simulink model "Model"  (R2024b)
settings: Solver=VariableStepAuto  StartTime=0.0  StopTime=30  MaxStep=0.001  RelTol=1e-4
PostLoadFcn:
  | SIM_setup
values from neighbouring files (symbols this model uses):
  A = 1.1    [RT14e_Parameters.m]    (also in RT15e_Parameters.m = 1.088; RT15evo_Parameters.m = 1.088; SIM_setup.m = 1.12)
  Aero_balance = 55    [RT14e_Parameters.m]    (also in RT15e_Parameters.m; RT15evo_Parameters.m; SIM_setup.m = 0.55)
  air_density = 1.29    [SIM_setup.m]
  Br_coef_of_friction_F = 0.33    [RT14e_Parameters.m]    (also in RT15e_Parameters.m; RT15evo_Parameters.m; SIM_setup.m = 0.25)
  Br_coef_of_friction_R = 0.33    [RT14e_Parameters.m]    (also in RT15e_Parameters.m; RT15evo_Parameters.m; SIM_setup.m = 0.25)
  Br_pistons_area_F = 3617.26/1e6    (= 0.00361726)    [RT14e_Parameters.m]    (also in RT15e_Parameters.m; RT15evo_Parameters.m; SIM_setup.m)
  Br_pistons_area_R = 2026.83/1e6    (= 0.00202683)    [RT14e_Parameters.m]    (also in RT15e_Parameters.m; RT15evo_Parameters.m; SIM_setup.m)
  Cd = 1.387    [SIM_setup.m]
  Cl = 3.299    [SIM_setup.m]
  CoG_z = 0.35    [RT14e_Parameters.m]    (also in RT15e_Parameters.m = 0.28495; RT15evo_Parameters.m = 0.28495; SIM_setup.m = 0.328)
  Default_Fz_F = g*(Mass*(Lr/Wheelbase))    [RT14e_Parameters.m]    (also in RT15e_Parameters.m; RT15evo_Parameters.m; SIM_setup.m = 608.22)
  Default_Fz_R = g*(Mass*(Lf/Wheelbase))    [RT14e_Parameters.m]    (also in RT15e_Parameters.m; RT15evo_Parameters.m; SIM_setup.m = 774.99)
  Effective_br_disk_r_F = 0.0905    [RT14e_Parameters.m]    (also in RT15e_Parameters.m; RT15evo_Parameters.m; SIM_setup.m)
  Effective_br_disk_r_R = 0.0895    [RT14e_Parameters.m]    (also in RT15e_Parameters.m; RT15evo_Parameters.m; SIM_setup.m)
  Fx = Data_Fx(2:end,3:end)    [RT14e_Parameters.m]    (also in RT15e_Parameters.m; RT15evo_Parameters.m; SIM_setup.m = Data_Fx(2:end,2:end))
  Fy = Data_Fy(2:end,3:end)    [RT14e_Parameters.m]    (also in RT15e_Parameters.m; RT15evo_Parameters.m; SIM_setup.m = Data_Fy(2:end,2:end))
  Fz = Data_Fy(2:end,2)    [RT14e_Parameters.m]    (also in RT15e_Parameters.m; RT15evo_Parameters.m; SIM_setup.m = Data_Fy(2:end,1))
  Half_track = 0.6    [SIM_setup.m]
  Iz_wehicle = 120    [RT14e_Parameters.m]    (also in RT15e_Parameters.m; RT15evo_Parameters.m; SIM_setup.m)
  Iz_wheel = 0.15    [RT14e_Parameters.m]    (also in RT15e_Parameters.m; RT15evo_Parameters.m; SIM_setup.m)
  Lateral_load_transfer_distribution = 0.55    [SIM_setup.m]
  Lf = Wheelbase - CoG_x    (= 0.77)    [RT14e_Parameters.m]    (also in RT15e_Parameters.m = 0.7504; RT15evo_Parameters.m = 0.7504; SIM_setup.m)
  Lr = Wheelbase - Lf    (= 0.755)    [RT14e_Parameters.m]    (also in RT15e_Parameters.m = 0.7746; RT15evo_Parameters.m = 0.7746; SIM_setup.m)
  Mass = Vehicle_mass + Driver_mass    (= 290)    [RT14e_Parameters.m]    (also in RT15e_Parameters.m = 265; RT15evo_Parameters.m; SIM_setup.m = 300)
  Max_Torque = 29.1    [SIM_setup.m]
  RB_torque_setting_1 = -2    [RT14e_Parameters.m]    (also in RT15e_Parameters.m; RT15evo_Parameters.m; SIM_setup.m)
  RB_torque_setting_10 = -20    [RT14e_Parameters.m]    (also in RT15e_Parameters.m; RT15evo_Parameters.m; SIM_setup.m)
  RB_torque_setting_2 = -4    [RT14e_Parameters.m]    (also in RT15e_Parameters.m; RT15evo_Parameters.m; SIM_setup.m)
  RB_torque_setting_3 = -6    [RT14e_Parameters.m]    (also in RT15e_Parameters.m; RT15evo_Parameters.m; SIM_setup.m)
  RB_torque_setting_4 = -8    [RT14e_Parameters.m]    (also in RT15e_Parameters.m; RT15evo_Parameters.m; SIM_setup.m)
  RB_torque_setting_5 = -10    [RT14e_Parameters.m]    (also in RT15e_Parameters.m; RT15evo_Parameters.m; SIM_setup.m)
  RB_torque_setting_6 = -12    [RT14e_Parameters.m]    (also in RT15e_Parameters.m; RT15evo_Parameters.m; SIM_setup.m)
  RB_torque_setting_7 = -14    [RT14e_Parameters.m]    (also in RT15e_Parameters.m; RT15evo_Parameters.m; SIM_setup.m)
  RB_torque_setting_8 = -16    [RT14e_Parameters.m]    (also in RT15e_Parameters.m; RT15evo_Parameters.m; SIM_setup.m)
  RB_torque_setting_9 = -18    [RT14e_Parameters.m]    (also in RT15e_Parameters.m; RT15evo_Parameters.m; SIM_setup.m)
  SA = Data_Fy(1,3:end)    [RT14e_Parameters.m]    (also in RT15e_Parameters.m; RT15evo_Parameters.m; SIM_setup.m = Data_Fy(1,2:end))
  SR = Data_Fx(1,3:end)    [RT14e_Parameters.m]    (also in RT15e_Parameters.m; RT15evo_Parameters.m; SIM_setup.m = Data_Fx(1,2:end))
  start_time = 182    [SIM_setup.m]
  start_velocity = Xsens_MTI_670_vel.Value(find(Xsens_MTI_670_vel.Time > start_time, 1)) * 1000 / 3600    [SIM_setup.m]
  Steering_angle_table = [0 9.9 19.9 30.14 40.57 51.05 61.29 70.87 79.38 91.9]    [SIM_setup.m]
  Steering_ratio_table = [3.25 3.24 3.23 3.20 3.16 3.10 3.04 2.97 2.90 2.77]    [SIM_setup.m]
  Tire_radius = 0.203    [RT14e_Parameters.m]    (also in RT15e_Parameters.m; RT15evo_Parameters.m; SIM_setup.m)
  Torque_limit_2 = Motor_maximum_torque*0.2    (= 5.82)    [RT14e_Parameters.m]    (also in RT15e_Parameters.m; RT15evo_Parameters.m; SIM_setup.m)
  Torque_limit_3 = Motor_maximum_torque*0.3    (= 8.73)    [RT14e_Parameters.m]    (also in RT15e_Parameters.m; RT15evo_Parameters.m; SIM_setup.m)
  Torque_limit_4 = Motor_maximum_torque*0.4    (= 11.64)    [RT14e_Parameters.m]    (also in RT15e_Parameters.m; RT15evo_Parameters.m; SIM_setup.m)
  Torque_limit_5 = Motor_maximum_torque*0.5    (= 14.55)    [RT14e_Parameters.m]    (also in RT15e_Parameters.m; RT15evo_Parameters.m; SIM_setup.m)
  Torque_limit_6 = Motor_maximum_torque*0.6    (= 17.46)    [RT14e_Parameters.m]    (also in RT15e_Parameters.m; RT15evo_Parameters.m; SIM_setup.m)
  Torque_limit_7 = Motor_maximum_torque*0.7    (= 20.37)    [RT14e_Parameters.m]    (also in RT15e_Parameters.m; RT15evo_Parameters.m; SIM_setup.m)
  Torque_limit_8 = Motor_maximum_torque*0.8    (= 23.28)    [RT14e_Parameters.m]    (also in RT15e_Parameters.m; RT15evo_Parameters.m; SIM_setup.m)
  Torque_limit_9 = 29.1    [RT14e_Parameters.m]    (also in RT15e_Parameters.m; RT15evo_Parameters.m; SIM_setup.m)
  Torque_limit_max = Motor_maximum_torque    (= 29.1)    [RT14e_Parameters.m]    (also in RT15e_Parameters.m; RT15evo_Parameters.m; SIM_setup.m)
  Torque_limit_min = Motor_maximum_torque*0.1    (= 2.91)    [RT14e_Parameters.m]    (also in RT15e_Parameters.m; RT15evo_Parameters.m; SIM_setup.m)
  Transmission_gear_ratio = 12.9    [SIM_setup.m]
  TV_RB_understeer_gradient_1 = -0.5    [RT14e_Parameters.m]    (also in RT15e_Parameters.m; RT15evo_Parameters.m; SIM_setup.m)
  TV_RB_understeer_gradient_10 = 0.005    [RT14e_Parameters.m]    (also in RT15e_Parameters.m; RT15evo_Parameters.m; SIM_setup.m)
  TV_RB_understeer_gradient_2 = -0.1    [RT14e_Parameters.m]    (also in RT15e_Parameters.m; RT15evo_Parameters.m; SIM_setup.m)
  TV_RB_understeer_gradient_3 = 0.08    [RT14e_Parameters.m]    (also in RT15e_Parameters.m; RT15evo_Parameters.m; SIM_setup.m)
  TV_RB_understeer_gradient_4 = 0.06    [RT14e_Parameters.m]    (also in RT15e_Parameters.m; RT15evo_Parameters.m; SIM_setup.m)
  TV_RB_understeer_gradient_5 = 0.05    [RT14e_Parameters.m]    (also in RT15e_Parameters.m; RT15evo_Parameters.m; SIM_setup.m)
  TV_RB_understeer_gradient_6 = 0.04    [RT14e_Parameters.m]    (also in RT15e_Parameters.m; RT15evo_Parameters.m; SIM_setup.m)
  TV_RB_understeer_gradient_7 = 0.03    [RT14e_Parameters.m]    (also in RT15e_Parameters.m; RT15evo_Parameters.m; SIM_setup.m)
  TV_RB_understeer_gradient_8 = 0.02    [RT14e_Parameters.m]    (also in RT15e_Parameters.m; RT15evo_Parameters.m; SIM_setup.m)
  TV_RB_understeer_gradient_9 = 0.01    [RT14e_Parameters.m]    (also in RT15e_Parameters.m; RT15evo_Parameters.m; SIM_setup.m)
  TV_understeer_gradient_1 = -0.5    [RT14e_Parameters.m]    (also in RT15e_Parameters.m; RT15evo_Parameters.m; SIM_setup.m)
  TV_understeer_gradient_10 = 0.002    [RT14e_Parameters.m]    (also in RT15e_Parameters.m; RT15evo_Parameters.m; SIM_setup.m)
  TV_understeer_gradient_2 = -0.1    [RT14e_Parameters.m]    (also in RT15e_Parameters.m; RT15evo_Parameters.m; SIM_setup.m)
  TV_understeer_gradient_3 = 0.06    [RT14e_Parameters.m]    (also in RT15e_Parameters.m; RT15evo_Parameters.m; SIM_setup.m)
  TV_understeer_gradient_4 = 0.05    [RT14e_Parameters.m]    (also in RT15e_Parameters.m; RT15evo_Parameters.m; SIM_setup.m)
  TV_understeer_gradient_5 = 0.04    [RT14e_Parameters.m]    (also in RT15e_Parameters.m; RT15evo_Parameters.m; SIM_setup.m)
  TV_understeer_gradient_6 = 0.03    [RT14e_Parameters.m]    (also in RT15e_Parameters.m; RT15evo_Parameters.m; SIM_setup.m)
  TV_understeer_gradient_7 = 0.02    [RT14e_Parameters.m]    (also in RT15e_Parameters.m; RT15evo_Parameters.m; SIM_setup.m)
  TV_understeer_gradient_8 = 0.01    [RT14e_Parameters.m]    (also in RT15e_Parameters.m; RT15evo_Parameters.m; SIM_setup.m)
  TV_understeer_gradient_9 = 0.005    [RT14e_Parameters.m]    (also in RT15e_Parameters.m; RT15evo_Parameters.m; SIM_setup.m)
  Wheel_base = 1.525    [SIM_setup.m]
  Wheel_rolling_resistance = 0.055    [RT14e_Parameters.m]    (also in RT15e_Parameters.m; RT15evo_Parameters.m; SIM_setup.m)
undefined symbols (not defined in the file or in its folder): Actual_Torque_Value_RL, Actual_Torque_Value_RR, aero_balance, APPS, Brake_Pressure_Front, Brake_Pressure_Rear, lateral_load_transfer_distribution, Steering_position, tire_radius, wheel_base, Xsens_MTI_670_accX, Xsens_MTI_670_accY, Xsens_MTI_670_gyrZ, Xsens_MTI_670_vel, Xsens_Yaw_Rate__deg_s_
libraries: simulink x20, simulink_extras x7, dspstat3 x4, slpidlib x1, slrealtimeloglib x1
(part 4 of 4)

== system Model/Drivetrain/TV Algorithm/Torque Vectoring/RB Yaw Rate Calculation/Understeer Gradeint Selection/Switch Case Action Subsystem20 ==
  Action Port : ActionPort  ActionPortLabel=case [ 9 ]:
  Constant : Constant  Value=TV_RB_understeer_gradient_9
  Out2 : Outport
  wires:
  Constant/1 -> Out2/1

== system Model/Drivetrain/TV Algorithm/Torque Vectoring/RB Yaw Rate Calculation/Understeer Gradeint Selection/Switch Case Action Subsystem21 ==
  Action Port : ActionPort  ActionPortLabel=case [ 10 ]:
  Constant : Constant  Value=TV_RB_understeer_gradient_10
  Out1 : Outport
  wires:
  Constant/1 -> Out1/1

== system Model/Drivetrain/TV Algorithm/Torque Vectoring/Yaw Rate Calculation/Understeer Gradeint Selection/Switch Case Action Subsystem ==
  Vehicle Speed [km/h] : Inport
  Action Port : ActionPort  ActionPortLabel=case [ 1 ]:
  1-D Lookup Table : Lookup_n-D  NumberOfTableDimensions=1  BreakpointsForDimension1=[25;30;35;40;45;50;55;60;65;70;75;80]  Table=[0.03;0.06;0.08;0.1;0.12;0.15;0.22;0.3;0.35;0.42;0.48;0.55]  InternalRulePriority=Speed  RndMeth=Simplest
  Saturation : Saturate  UpperLimit=80  LowerLimit=25
  Saturation1 : Saturate  UpperLimit=0.55  LowerLimit=0.03
  Out1 : Outport
  wires:
  1-D Lookup Table/1 -> Saturation1/1
  Saturation1/1 -> Out1/1
  Vehicle Speed [km/h]/1 -> Saturation/1
  Saturation/1 -> 1-D Lookup Table/1

== system Model/Drivetrain/TV Algorithm/Torque Vectoring/Yaw Rate Calculation/Understeer Gradeint Selection/Switch Case Action Subsystem1 ==
  Vehicle Speed [km/h] : Inport
  Action Port : ActionPort  ActionPortLabel=case [ 2 ]:
  1-D Lookup Table : Lookup_n-D  NumberOfTableDimensions=1  BreakpointsForDimension1=[25;30;35;40;45;50;55;60;65;70;75;80]  Table=[0.02;0.04;0.06;0.08;0.1;0.14;0.16;0.2;0.25;0.32;0.38;0.45]  InternalRulePriority=Speed  RndMeth=Simplest
  Saturation : Saturate  UpperLimit=80  LowerLimit=25
  Saturation1 : Saturate  UpperLimit=0.45  LowerLimit=0.02
  Out1 : Outport
  wires:
  Vehicle Speed [km/h]/1 -> Saturation/1
  Saturation/1 -> 1-D Lookup Table/1
  1-D Lookup Table/1 -> Saturation1/1
  Saturation1/1 -> Out1/1

== system Model/Drivetrain/TV Algorithm/Torque Vectoring/Yaw Rate Calculation/Understeer Gradeint Selection/Switch Case Action Subsystem10 ==
  Vehicle Speed [km/h] : Inport
  Action Port : ActionPort  ActionPortLabel=default:
  1-D Lookup Table : Lookup_n-D  NumberOfTableDimensions=1  BreakpointsForDimension1=[25;30;35;40;45;50;55;60;65;70;75;80]  Table=[0.003;0.005;0.008;0.01;0.03;0.05;0.08;0.12;0.15;0.18;0.25;0.3]  InternalRulePriority=Speed  RndMeth=Simplest
  Saturation : Saturate  UpperLimit=80  LowerLimit=25
  Saturation1 : Saturate  UpperLimit=0.3  LowerLimit=0.001
  Out1 : Outport
  wires:
  1-D Lookup Table/1 -> Saturation1/1
  Vehicle Speed [km/h]/1 -> Saturation/1
  Saturation1/1 -> Out1/1
  Saturation/1 -> 1-D Lookup Table/1

== system Model/Drivetrain/TV Algorithm/Torque Vectoring/Yaw Rate Calculation/Understeer Gradeint Selection/Switch Case Action Subsystem11 ==
  Action Port : ActionPort  ActionPortLabel=case [ 1 ]:
  Constant1 : Constant  Value=TV_understeer_gradient_1
  Out1 : Outport
  wires:
  Constant1/1 -> Out1/1

== system Model/Drivetrain/TV Algorithm/Torque Vectoring/Yaw Rate Calculation/Understeer Gradeint Selection/Switch Case Action Subsystem12 ==
  Action Port : ActionPort  ActionPortLabel=case [ 2 ]:
  Constant : Constant  Value=TV_understeer_gradient_2
  Out2 : Outport
  wires:
  Constant/1 -> Out2/1

== system Model/Drivetrain/TV Algorithm/Torque Vectoring/Yaw Rate Calculation/Understeer Gradeint Selection/Switch Case Action Subsystem13 ==
  Action Port : ActionPort  ActionPortLabel=default:
  Constant : Constant  Value=TV_understeer_gradient_8
  Out2 : Outport
  wires:
  Constant/1 -> Out2/1

== system Model/Drivetrain/TV Algorithm/Torque Vectoring/Yaw Rate Calculation/Understeer Gradeint Selection/Switch Case Action Subsystem14 ==
  Action Port : ActionPort  ActionPortLabel=case [ 3 ]:
  Constant1 : Constant  Value=TV_understeer_gradient_3
  Out1 : Outport
  wires:
  Constant1/1 -> Out1/1

== system Model/Drivetrain/TV Algorithm/Torque Vectoring/Yaw Rate Calculation/Understeer Gradeint Selection/Switch Case Action Subsystem15 ==
  Action Port : ActionPort  ActionPortLabel=case [ 4 ]:
  Constant : Constant  Value=TV_understeer_gradient_4
  Out2 : Outport
  wires:
  Constant/1 -> Out2/1

== system Model/Drivetrain/TV Algorithm/Torque Vectoring/Yaw Rate Calculation/Understeer Gradeint Selection/Switch Case Action Subsystem16 ==
  Action Port : ActionPort  ActionPortLabel=case [ 5 ]:
  Constant : Constant  Value=TV_understeer_gradient_5
  Out1 : Outport
  wires:
  Constant/1 -> Out1/1

== system Model/Drivetrain/TV Algorithm/Torque Vectoring/Yaw Rate Calculation/Understeer Gradeint Selection/Switch Case Action Subsystem17 ==
  Action Port : ActionPort  ActionPortLabel=case [ 6 ]:
  Constant : Constant  Value=TV_understeer_gradient_6
  Out2 : Outport
  wires:
  Constant/1 -> Out2/1

== system Model/Drivetrain/TV Algorithm/Torque Vectoring/Yaw Rate Calculation/Understeer Gradeint Selection/Switch Case Action Subsystem18 ==
  Action Port : ActionPort  ActionPortLabel=case [ 7 ]:
  Constant : Constant  Value=TV_understeer_gradient_7
  Out1 : Outport
  wires:
  Constant/1 -> Out1/1

== system Model/Drivetrain/TV Algorithm/Torque Vectoring/Yaw Rate Calculation/Understeer Gradeint Selection/Switch Case Action Subsystem19 ==
  Action Port : ActionPort  ActionPortLabel=case [ 8 ]:
  Constant : Constant  Value=TV_understeer_gradient_8
  Out2 : Outport
  wires:
  Constant/1 -> Out2/1

== system Model/Drivetrain/TV Algorithm/Torque Vectoring/Yaw Rate Calculation/Understeer Gradeint Selection/Switch Case Action Subsystem2 ==
  Vehicle Speed [km/h] : Inport
  Action Port : ActionPort  ActionPortLabel=case [ 3 ]:
  1-D Lookup Table1 : Lookup_n-D  NumberOfTableDimensions=1  BreakpointsForDimension1=[25;30;35;40;45;50;55;60;65;70;75;80]  Table=[0.01;0.02;0.04;0.06;0.08;0.12;0.16;0.22;0.28;0.35;0.42;0.5]  InternalRulePriority=Speed  RndMeth=Simplest
  Saturation2 : Saturate  UpperLimit=80  LowerLimit=25
  Saturation3 : Saturate  LowerLimit=0.01
  Out1 : Outport
  wires:
  Vehicle Speed [km/h]/1 -> Saturation2/1
  Saturation3/1 -> Out1/1
  Saturation2/1 -> 1-D Lookup Table1/1
  1-D Lookup Table1/1 -> Saturation3/1

== system Model/Drivetrain/TV Algorithm/Torque Vectoring/Yaw Rate Calculation/Understeer Gradeint Selection/Switch Case Action Subsystem20 ==
  Action Port : ActionPort  ActionPortLabel=case [ 9 ]:
  Constant : Constant  Value=TV_understeer_gradient_9
  Out2 : Outport
  wires:
  Constant/1 -> Out2/1

== system Model/Drivetrain/TV Algorithm/Torque Vectoring/Yaw Rate Calculation/Understeer Gradeint Selection/Switch Case Action Subsystem21 ==
  Action Port : ActionPort  ActionPortLabel=case [ 10 ]:
  Constant : Constant  Value=TV_understeer_gradient_10
  Out1 : Outport
  wires:
  Constant/1 -> Out1/1

== system Model/Drivetrain/TV Algorithm/Torque Vectoring/Yaw Rate Calculation/Understeer Gradeint Selection/Switch Case Action Subsystem3 ==
  Vehicle Speed [km/h] : Inport
  Action Port : ActionPort  ActionPortLabel=case [ 4 ]:
  1-D Lookup Table : Lookup_n-D  NumberOfTableDimensions=1  BreakpointsForDimension1=[25;30;35;40;45;50;55;60;65;70;75;80]  Table=[0.005;0.02;0.04;0.06;0.08;0.1;0.12;0.15;0.18;0.25;0.32;0.4]  InternalRulePriority=Speed  RndMeth=Simplest
  Saturation : Saturate  UpperLimit=80  LowerLimit=25
  Saturation1 : Saturate  UpperLimit=0.4  LowerLimit=0.005
  Out1 : Outport
  wires:
  Vehicle Speed [km/h]/1 -> Saturation/1
  Saturation1/1 -> Out1/1
  1-D Lookup Table/1 -> Saturation1/1
  Saturation/1 -> 1-D Lookup Table/1

== system Model/Drivetrain/TV Algorithm/Torque Vectoring/Yaw Rate Calculation/Understeer Gradeint Selection/Switch Case Action Subsystem4 ==
  Vehicle Speed [km/h] : Inport
  Action Port : ActionPort  ActionPortLabel=case [ 5 ]:
  1-D Lookup Table : Lookup_n-D  NumberOfTableDimensions=1  BreakpointsForDimension1=[25;30;35;40;45;50;55;60;65;70;75;80]  Table=[0.003;0.006;0.01;0.03;0.06;0.08;0.1;0.13;0.16;0.2;0.28;0.35]  InternalRulePriority=Speed  RndMeth=Simplest
  Saturation : Saturate  UpperLimit=80  LowerLimit=25
  Saturation1 : Saturate  UpperLimit=0.35  LowerLimit=0.003
  Out1 : Outport
  wires:
  1-D Lookup Table/1 -> Saturation1/1
  Vehicle Speed [km/h]/1 -> Saturation/1
  Saturation1/1 -> Out1/1
  Saturation/1 -> 1-D Lookup Table/1

== system Model/Drivetrain/TV Algorithm/Torque Vectoring/Yaw Rate Calculation/Understeer Gradeint Selection/Switch Case Action Subsystem5 ==
  Vehicle Speed [km/h] : Inport
  Action Port : ActionPort  ActionPortLabel=case [ 6 ]:
  1-D Lookup Table : Lookup_n-D  NumberOfTableDimensions=1  BreakpointsForDimension1=[25;30;35;40;45;50;55;60;65;70;75;80]  Table=[0.003;0.005;0.008;0.01;0.03;0.05;0.08;0.12;0.15;0.18;0.25;0.3]  InternalRulePriority=Speed  RndMeth=Simplest
  Saturation : Saturate  UpperLimit=80  LowerLimit=25
  Saturation1 : Saturate  UpperLimit=0.3  LowerLimit=0.003
  Out1 : Outport
  wires:
  Saturation/1 -> 1-D Lookup Table/1
  Saturation1/1 -> Out1/1
  1-D Lookup Table/1 -> Saturation1/1
  Vehicle Speed [km/h]/1 -> Saturation/1

== system Model/Drivetrain/TV Algorithm/Torque Vectoring/Yaw Rate Calculation/Understeer Gradeint Selection/Switch Case Action Subsystem6 ==
  Vehicle Speed [km/h] : Inport
  Action Port : ActionPort  ActionPortLabel=case [ 7 ]:
  1-D Lookup Table : Lookup_n-D  NumberOfTableDimensions=1  BreakpointsForDimension1=[25;30;35;40;45;50;55;60;65;70;75;80]  Table=[0.002;0.003;0.005;0.008;0.01;0.03;0.06;0.09;0.12;0.16;0.2;0.25]  InternalRulePriority=Speed  RndMeth=Simplest
  Saturation : Saturate  UpperLimit=80  LowerLimit=25
  Saturation1 : Saturate  UpperLimit=0.25  LowerLimit=0.002
  Out1 : Outport
  wires:
  Vehicle Speed [km/h]/1 -> Saturation/1
  Saturation1/1 -> Out1/1
  Saturation/1 -> 1-D Lookup Table/1
  1-D Lookup Table/1 -> Saturation1/1

== system Model/Drivetrain/TV Algorithm/Torque Vectoring/Yaw Rate Calculation/Understeer Gradeint Selection/Switch Case Action Subsystem7 ==
  Vehicle Speed [km/h] : Inport
  Action Port : ActionPort  ActionPortLabel=case [ 8 ]:
  1-D Lookup Table : Lookup_n-D  NumberOfTableDimensions=1  BreakpointsForDimension1=[25;30;35;40;45;50;55;60;65;70;75;80]  Table=[0.001;0.002;0.005;0.007;0.008;0.015;0.03;0.06;0.08;0.12;0.15;0.2]  InternalRulePriority=Speed  RndMeth=Simplest
  Saturation : Saturate  UpperLimit=80  LowerLimit=25
  Saturation1 : Saturate  UpperLimit=0.2  LowerLimit=0.001
  Out1 : Outport
  wires:
  Saturation1/1 -> Out1/1
  1-D Lookup Table/1 -> Saturation1/1
  Saturation/1 -> 1-D Lookup Table/1
  Vehicle Speed [km/h]/1 -> Saturation/1

== system Model/Drivetrain/TV Algorithm/Torque Vectoring/Yaw Rate Calculation/Understeer Gradeint Selection/Switch Case Action Subsystem8 ==
  Vehicle Speed [km/h] : Inport
  Action Port : ActionPort  ActionPortLabel=case [ 9 ]:
  1-D Lookup Table : Lookup_n-D  NumberOfTableDimensions=1  BreakpointsForDimension1=[25;30;35;40;45;50;55;60;65;70;75;80]  Table=[0.001;0.002;0.005;0.007;0.008;0.009;0.01;0.02;0.03;0.04;0.07;0.1]  InternalRulePriority=Speed  RndMeth=Simplest
  Saturation : Saturate  UpperLimit=80  LowerLimit=25
  Saturation1 : Saturate  UpperLimit=0.12  LowerLimit=0.001
  Out1 : Outport
  wires:
  Vehicle Speed [km/h]/1 -> Saturation/1
  Saturation1/1 -> Out1/1
  Saturation/1 -> 1-D Lookup Table/1
  1-D Lookup Table/1 -> Saturation1/1

== system Model/Drivetrain/TV Algorithm/Torque Vectoring/Yaw Rate Calculation/Understeer Gradeint Selection/Switch Case Action Subsystem9 ==
  Vehicle Speed [km/h] : Inport
  Action Port : ActionPort  ActionPortLabel=case [ 10 ]:
  1-D Lookup Table1 : Lookup_n-D  NumberOfTableDimensions=1  BreakpointsForDimension1=[25;30;35;40;45;50;55;60;65;70;75;80]  Table=[0.001;0.003;0.007;0.009;0.01;0.013;0.018;0.022;0.03;0.04;0.07;0.1]  InternalRulePriority=Speed  RndMeth=Simplest
  Saturation : Saturate  UpperLimit=80  LowerLimit=25
  Saturation2 : Saturate  UpperLimit=0.1  LowerLimit=0.001
  Out1 : Outport
  wires:
  Vehicle Speed [km/h]/1 -> Saturation/1
  Saturation/1 -> 1-D Lookup Table1/1
  Saturation2/1 -> Out1/1
  1-D Lookup Table1/1 -> Saturation2/1
